simulink model "ModeloBloqueTank02"  (R2013a)
settings: Solver=ode45  StartTime=0.0  StopTime=10.0  RelTol=1e-3
settings Model: Creator=Cristhian Ivan  LastModifiedBy=Cristhian Ivan

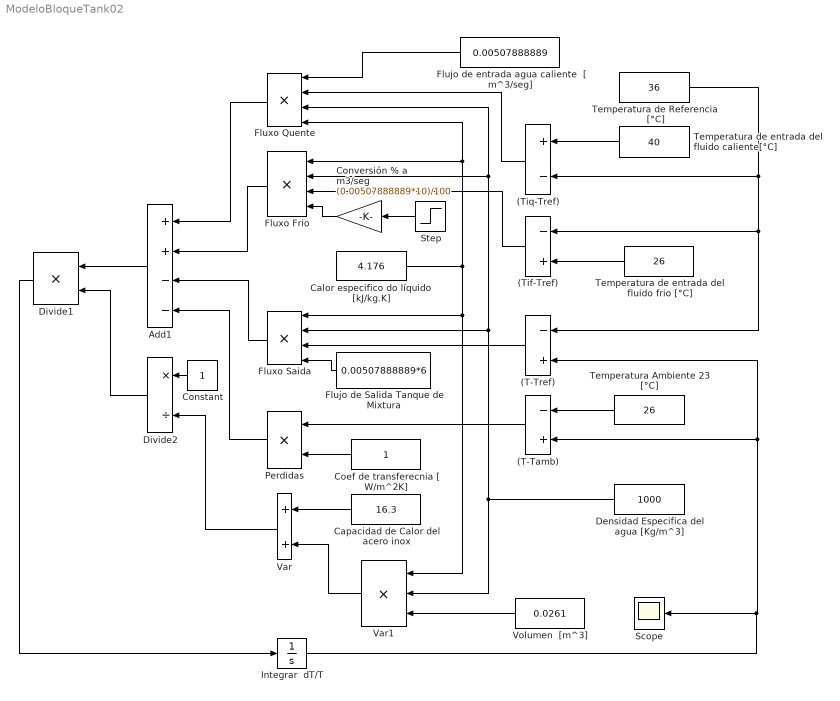
== system ModeloBloqueTank02 ==
  (T-Tamb) : Sum  Inputs=-+
  (T-Tref) : Sum  Inputs=-+
  (Tif-Tref) : Sum  Inputs=-+
  (Tiq-Tref) : Sum  Inputs=+-
  Add1 : Sum  Inputs=++--
  Calor especifico do líquido  [kJ/kg.K] : Constant  Value=4.176
  "Capacidad de Calor del acero inox " : Constant  Value=16.3
  Coef de transferecnia [ W/m^2K] : Constant
  Constant : Constant
  Conversión % a m3/seg : Gain  Gain=(0.00507888889*10)/100
  "Densidad Especifica del agua [Kg/m^3] " : Constant  Value=1000
  Divide1 : Product  Inputs=**
  Divide2 : Product  Inputs=*/
  "Flujo de Salida Tanque de Mixtura " : Constant  Value=0.00507888889*6
  Flujo de entrada agua caliente  [ m^3/seg] : Constant  Value=0.00507888889
  Fluxo Frio : Product  Inputs=****
  Fluxo Quente : Product  Inputs=****
  Fluxo Saida : Product  Inputs=****
  Integrar  dT/T : Integrator
  Perdidas : Product  Inputs=**
  Scope : Scope
      settings: TimeRange=10  YMin=58.165  YMax=58.225
  Step : Step  Time=0  After=5  SampleTime=0
  "Temperatura Ambiente 23 [°C] " : Constant  Value=26
  Temperatura de Referencia  [°C] : Constant  Value=36
  Temperatura de entrada del fluido caliente[°C] : Constant  Value=40
  Temperatura de entrada del fluido frio [°C] : Constant  Value=26
  Var : Sum
  Var1 : Product  Inputs=***
  Volumen  [m^3] : Constant  Value=0.0261
  wires:
  Add1/1 -> Divide1/1
  Fluxo Quente/1 -> Add1/1
  Temperatura de entrada del fluido caliente[°C]/1 -> (Tiq-Tref)/1
  Calor especifico do líquido  [kJ/kg.K]/1 -> Fluxo Saida/1, Var1/1, Fluxo Quente/4, Fluxo Frio/1
  "Densidad Especifica del agua [Kg/m^3] "/1 -> Fluxo Quente/3, Fluxo Frio/2, Fluxo Saida/2, Var1/2
  "Capacidad de Calor del acero inox "/1 -> Var/1
  Var1/1 -> Var/2
  Volumen  [m^3]/1 -> Var1/3
  Step/1 -> Conversión % a m3/seg/1
  Conversión % a m3/seg/1 -> Fluxo Frio/4
  Fluxo Frio/1 -> Add1/2
  Temperatura de Referencia  [°C]/1 -> (T-Tref)/1, (Tif-Tref)/1, (Tiq-Tref)/2
  Divide1/1 -> Integrar  dT/T/1
  Integrar  dT/T/1 -> (T-Tref)/2, (T-Tamb)/2, Scope/1
  (T-Tref)/1 -> Fluxo Saida/3
  "Flujo de Salida Tanque de Mixtura "/1 -> Fluxo Saida/4
  Flujo de entrada agua caliente  [ m^3/seg]/1 -> Fluxo Quente/1
  Fluxo Saida/1 -> Add1/3
  Perdidas/1 -> Add1/4
  Coef de transferecnia [ W/m^2K]/1 -> Perdidas/2
  "Temperatura Ambiente 23 [°C] "/1 -> (T-Tamb)/1
  (T-Tamb)/1 -> Perdidas/1
  (Tif-Tref)/1 -> Fluxo Frio/3
  Temperatura de entrada del fluido frio [°C]/1 -> (Tif-Tref)/2
  Divide2/1 -> Divide1/2
  Constant/1 -> Divide2/1
  Var/1 -> Divide2/2
  (Tiq-Tref)/1 -> Fluxo Quente/2
